simulink model "Synch_Machine_Simple"  (R2022b)
settings: Solver=ode23tb  StartTime=0.0  StopTime=10  RelTol=1e-3  EnableMultiTasking=on
PostLoadFcn:
  | warning off Simulink:Engine:UsingDefaultMaxStepSize
libraries: spsThreePhaseSeriesRLCLoadLib x1, spsSimplifiedSynchronousMachineSIUnitsLib x1, spsThreePhaseVIMeasurementLib x1, spspowerguiLib x1
Description:
  | Copyright 2014-2022 The MathWorks, Inc.
settings Model: Creator=smiller  LastModifiedBy=smiller
settings SolverCC: AlgebraicLoopSolver=TrustRegion
settings DataIOCC: LimitDataPoints=on  SaveFormat=Array  ReturnWorkspaceOutputs=off
settings OptimizationCC: LifeSpan=inf
settings DebuggingCC: UnderspecifiedInitializationDetection=Classic  MergeDetectMultiDrivingBlocksExec=none  SolverPrmCheckMsg=warning  UnconnectedInputMsg=warning  UnconnectedOutputMsg=warning  UnconnectedLineMsg=warning  AllowSymbolicDim=off  StateNameClashWarn=warning  PregeneratedLibrarySubsystemCodeDiagnostic=none  SFUnexpectedBacktrackingDiag=warning  SFNoUnconditionalDefaultTransitionDiag=warning  SFExecutionAtInitializationDiag=none  SFMachineParentedDataDiag=warning  ArithmeticOperatorsInVariantConditions=warning
settings HardwareCC: ProdBitPerPointer=32  ProdBitPerSizeT=32  ProdBitPerPtrDiffT=32  ProdLargestAtomicFloat=None  ProdIntDivRoundTo=Undefined  ProdEndianess=Unspecified  ProdWordSize=32  ProdHWDeviceType=32-bit Generic
settings ModelReferenceCC: EnableRefExpFcnMdlSchedulingChecks=on  PropagateSignalLabelsOutOfModel=off
settings SFSimCC: SimUseLocalCustomCode=off  CustomCodeUndefinedFunction=UseInterfaceOnly
settings RTWCC: RTWUseLocalCustomCode=off  DLArmComputeVersion=19.05
settings CodeAppCC: StateflowObjectComments=on
settings GRTTargetCC: TargetLangStandard=C89/C90 (ANSI)
settings ConfigComp: CovMetricSettings=dw  CovSaveCumulativeToWorkspaceVar=on  CovSaveSingleToWorkspaceVar=on  CovExternalEMLEnable=off  CovSFcnEnable=off
settings SimscapeCC: SimscapeNormalizeSystem=off  SimscapeNominalValues="[{\"value\":\"10\",\"unit\":\"V\"},{\"value\":\"1\",\"unit\":\"A\"},{\"value\":\"10\",\"unit\":\"N*m\"},{\"value\":\"10\",\"unit\":\"bar\"},{\"value\":\"100\",\"unit\":\"kJ/kg\"},{\"value\":\"1\",\"unit\":\"kW\"},{\"value\":\"300\",\"unit\":\"K\"},{\"value\":\"100\",\"unit\":\"cm^3/s\"},{\"value\":\"1\",\"unit\":\"kN\"},{\"value\":\"1\",\"unit\":\"g/cm^3\"},{\"value\":\"1\",\"unit\":\"l\"},{\"value\":\"1\",\"unit\":\"cm^2\"},{\"value\":\"60\",\"unit\":\"Hz\"}]"

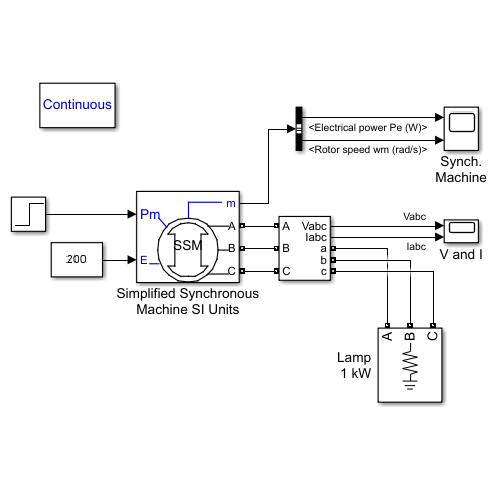
[thumbnail: Simulink's stored preview of the top-level diagram]
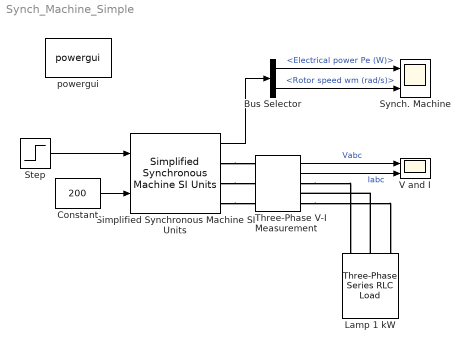
== system Synch_Machine_Simple ==
  Bus Selector : BusSelector  OutputSignals=Electrical power Pe (W),Rotor speed wm (rad/s)
  Constant : Constant  Value=200
  Lamp 1 kW : spsThreePhaseSeriesRLCLoadLib/Three-Phase Series RLC Load  LConnTagsString=A|B|C  Configuration=Y (grounded)  NominalVoltage=(200)*1  Vabc=[1e3 1e3 1e3]  Vabcp=[1e3 1e3 1e3]  NominalFrequency=400  UnbalancedPower=off  ActivePower=1e3  InductivePower=0  CapacitivePower=0  Pabc=[10e3 9e3 11e3]  QLabc=[100 90 110]  QCabc=[100 90 110]  Pabcp=[10e3 9e3 11e3]  QLabcp=[100 90 110]  QCabcp=[100 90 110]  Measurements=None  LoadType=constant PQ
  Simplified Synchronous Machine SI Units : spsSimplifiedSynchronousMachineSIUnitsLib/Simplified Synchronous Machine SI Units  ConnectionType=3-wire Y  MechanicalLoad=Mechanical power Pm  MeasurementBus=off  NominalParameters=[50e3 200 400]  Mechanical="[0.2,  10,  2]"  InternalRL="[0.0204  0.8104e-3]"  InitialConditions=[0 0 0 0 0 0 0 0]  IterativeDiscreteModel=Trapezoidal non iterative  TsBlock=-1  TsPowergui=0  LoadFlowParameters=[1 0 0 0 0]  Units=1  BusType=swing  Pref=0  Qref=0  Qmin=-inf  Qmax=+inf  PLF=0  QLF=0
  Step : Step  Time=5  After=50e3  SampleTime=0
  Synch. Machine : Scope  NumInputPorts=2
  Three-Phase V-I Measurement : spsThreePhaseVIMeasurementLib/Three-Phase V-I Measurement  VoltageMeasurement=phase-to-ground  SetLabelV=off  LabelV=Vabc  Vpu=off  VpuLL=off  CurrentMeasurement=yes  SetLabelI=off  LabelI=Iabc  Ipu=off  Pbase=100e6  Vbase=500e3  OutputType=Complex  PhasorSimulation=off  PSBequivalent=0
  V and I : Scope  NumInputPorts=2
  powergui : spspowerguiLib/powergui  Priority=1  SimulationMode=Continuous  SampleTime=50e-6  frequency=60  Iterations=50  frequencyindice=400  Pbase=100e6  ErrMax=0.0001  UnitsV=kV  UnitsW=MW  buscounter=0  FunctionMessages=off  echomessages=off  EnableUseOfTLC=off  CurrentSourceSwitches=on  DisableSnubberDevices=off  DisableRonSwitches=off  DisableVfSwitches=off  DisplayEquations=off  AutomaticDiscreteSolvers=off  SolverType=Tustin  Interpol=off  ExternalGateDelay=off  methode=off  Ts=0  x0status=blocks  SPID=off  SwTol=0  HookPort=off  NonlinearTolerance=0  nMaxIteration=15  ContinueOnMaxIteration=off  RestoreLinks=warning  ResistiveCurrentMeasurement=off  Frange=[0:2:500]  Ylog=off  Xlog=on  ShowGrid=off  save=off  variable=ZData  structure=0  ZoomFFT=off  StartTime=0.0  cycles=1  DisplayStyle=1  fundamental=60  FreqAxis=off  MaxFrequency=1000  frequencyindicesteady=1  RmsSteady=1  display=off
  wires:
  Constant/1 -> Simplified Synchronous Machine SI Units/2
  Step/1 -> Simplified Synchronous Machine SI Units/1
  Simplified Synchronous Machine SI Units/1 -> Bus Selector/1
  Bus Selector/2 -> Synch. Machine/2  "<Rotor speed wm (rad/s)>"
  Bus Selector/1 -> Synch. Machine/1  "<Electrical power Pe (W)>"
  Three-Phase V-I Measurement/1 -> V and I/1  "Vabc"
  Three-Phase V-I Measurement/2 -> V and I/2  "Iabc"
  connections:
  Simplified Synchronous Machine SI Units/RConn2 -- Three-Phase V-I Measurement/LConn2
  Simplified Synchronous Machine SI Units/RConn1 -- Three-Phase V-I Measurement/LConn1
  Simplified Synchronous Machine SI Units/RConn3 -- Three-Phase V-I Measurement/LConn3
  Three-Phase V-I Measurement/RConn1 -- Lamp 1 kW/LConn1
  Lamp 1 kW/LConn2 -- Three-Phase V-I Measurement/RConn2
  Three-Phase V-I Measurement/RConn3 -- Lamp 1 kW/LConn3
